simulink model "sim_battery_pack_simulink_18_11"  (R2021a)
settings: Solver=FixedStepAuto  StartTime=0.0  StopTime=3460.480  FixedStep=0.01  RelTol=1e-3
values from neighbouring files (symbols this model uses):
  Af = 1.4*1.6    (= 2.24)    [battery_pack_init_18_11.m]
  b = 0.002    [battery_pack_init_18_11.m]
  Batt_Eff = .98    (= 0.98)    [battery_pack_init_18_11.m]
  Batt_Ene_Cap = 7.37    [battery_pack_init_18_11.m]
  cd = 0.45    [battery_pack_init_18_11.m]
  dt = 0.01    [battery_pack_init_18_11.m]
  g = 9.81    [battery_pack_init_18_11.m]
  Gr = 5.75*.85    (= 4.8875)    [battery_pack_init_18_11.m]
  Grade = 7    [battery_pack_init_18_11.m]
  Ini_SOC = 100    [battery_pack_init_18_11.m]
  kappa = 0.1    [battery_pack_init_18_11.m]
  M = M_k+M_P    (= 445)    [battery_pack_init_18_11.m]
  M_Trq = T_m    [battery_pack_init_18_11.m]
  M_w = w_m    [battery_pack_init_18_11.m]
  Mot_Eff = .9    (= 0.9)    [battery_pack_init_18_11.m]
  mu = 0.016    [battery_pack_init_18_11.m]
  Np = 7    [battery_pack_init_18_11.m]
  Ns = 12    [battery_pack_init_18_11.m]
  Qgain = 1    [battery_pack_init_18_11.m]
  R0 = zeros(numpoles,1)    [battery_pack_init_18_11.m]
  R0Param = getParamESC('R0Param',T,cell_model)    [battery_pack_init_18_11.m]
  R_w = .3048/2    (= 0.1524)    [battery_pack_init_18_11.m]
  Re_spe_max = 50*5/18    (= 13.8888888889)    [battery_pack_init_18_11.m]
  Re_spe_min = 0*5/18    (= 0)    [battery_pack_init_18_11.m]
  rho = 1.225    [battery_pack_init_18_11.m]
  rt = .0008    (= 0.0008)    [battery_pack_init_18_11.m]
  T = 40    [battery_pack_init_18_11.m]
  T_MIDC = T_MIDC(1:72)    [battery_pack_init_18_11.m]
  Trans_Eff = .95    (= 0.95)    [battery_pack_init_18_11.m]
  V_MIDC = V_MIDC(1:72)    [battery_pack_init_18_11.m]
  Z0 = 0.75 + (1-0.75).*rand(1,Np)    [battery_pack_init_18_11.m]
undefined symbols (not defined in the file or in its folder): cell_model, FLbattery, gain, iload, sigbuilder_block, VMIDC
libraries: simulink x16, autolibshared x2, pid_lib x1, simulink_extras x1
(part 3 of 17)

== system sim_battery_pack_simulink_18_11/SCM7/cell6 ==
  ik1 : Inport
  Constant : Constant  Value=R0
  Constant1 : Constant  Value=dt
  Constant2 : Constant  Value=T
  States : Scope  NumInputPorts=2
  Unit Delay : UnitDelay  InitialCondition=Z0(6,7)  SampleTime=-1  HasFrameUpgradeWarning=on
  Unit Delay1 : UnitDelay  SampleTime=-1  HasFrameUpgradeWarning=on
  Voltage : Scope  NumInputPorts=2
  cell_model : MATLAB Function  TreatAsAtomicUnit=on
  V1 : Outport
  Z1 : Outport  Port=2
  irc1 : Outport  Port=3
  wires:
  cell_model/4(OCV) -> Voltage/2
  ik1/1 -> cell_model/6(ik)
  cell_model/3(zkc) -> Z1/1, Unit Delay/1, States/1
  cell_model/1(vk) -> V1/1, Voltage/1
  Constant1/1 -> cell_model/2(deltaT)
  Constant2/1 -> cell_model/1(T)
  Unit Delay/1 -> cell_model/4(zkp)
  cell_model/2(irkc) -> irc1/1, Unit Delay1/1, States/2
  Unit Delay1/1 -> cell_model/5(irkp)
  Constant/1 -> cell_model/3(iR0)

== system sim_battery_pack_simulink_18_11/SCM7/cell7 ==
  ik1 : Inport
  Constant : Constant  Value=R0
  Constant1 : Constant  Value=dt
  Constant2 : Constant  Value=T
  States : Scope  NumInputPorts=2
  Unit Delay : UnitDelay  InitialCondition=Z0(7,7)  SampleTime=-1  HasFrameUpgradeWarning=on
  Unit Delay1 : UnitDelay  SampleTime=-1  HasFrameUpgradeWarning=on
  Voltage : Scope  NumInputPorts=2
  cell_model : MATLAB Function  TreatAsAtomicUnit=on
  V1 : Outport
  Z1 : Outport  Port=2
  irc1 : Outport  Port=3
  wires:
  Constant/1 -> cell_model/3(iR0)
  Unit Delay1/1 -> cell_model/5(irkp)
  cell_model/2(irkc) -> States/2, Unit Delay1/1, irc1/1
  Unit Delay/1 -> cell_model/4(zkp)
  Constant2/1 -> cell_model/1(T)
  Constant1/1 -> cell_model/2(deltaT)
  cell_model/1(vk) -> Voltage/1, V1/1
  cell_model/3(zkc) -> States/1, Unit Delay/1, Z1/1
  ik1/1 -> cell_model/6(ik)
  cell_model/4(OCV) -> Voltage/2

== system sim_battery_pack_simulink_18_11/SCM7/cell8 ==
  ik1 : Inport
  Constant : Constant  Value=R0
  Constant1 : Constant  Value=dt
  Constant2 : Constant  Value=T
  States : Scope  NumInputPorts=2
  Unit Delay : UnitDelay  InitialCondition=Z0(8,7)  SampleTime=-1  HasFrameUpgradeWarning=on
  Unit Delay1 : UnitDelay  SampleTime=-1  HasFrameUpgradeWarning=on
  Voltage : Scope  NumInputPorts=2
  cell_model : MATLAB Function  TreatAsAtomicUnit=on
  V1 : Outport
  Z1 : Outport  Port=2
  irc1 : Outport  Port=3
  wires:
  cell_model/4(OCV) -> Voltage/2
  ik1/1 -> cell_model/6(ik)
  cell_model/3(zkc) -> Z1/1, Unit Delay/1, States/1
  cell_model/1(vk) -> V1/1, Voltage/1
  Constant1/1 -> cell_model/2(deltaT)
  Constant2/1 -> cell_model/1(T)
  Unit Delay/1 -> cell_model/4(zkp)
  cell_model/2(irkc) -> irc1/1, Unit Delay1/1, States/2
  Unit Delay1/1 -> cell_model/5(irkp)
  Constant/1 -> cell_model/3(iR0)

== system sim_battery_pack_simulink_18_11/SCM7/cell9 ==
  ik1 : Inport
  Constant : Constant  Value=R0
  Constant1 : Constant  Value=dt
  Constant2 : Constant  Value=T
  States : Scope  NumInputPorts=2
  Unit Delay : UnitDelay  InitialCondition=Z0(9,7)  SampleTime=-1  HasFrameUpgradeWarning=on
  Unit Delay1 : UnitDelay  SampleTime=-1  HasFrameUpgradeWarning=on
  Voltage : Scope  NumInputPorts=2
  cell_model : MATLAB Function  TreatAsAtomicUnit=on
  V1 : Outport
  Z1 : Outport  Port=2
  irc1 : Outport  Port=3
  wires:
  Constant/1 -> cell_model/3(iR0)
  Unit Delay1/1 -> cell_model/5(irkp)
  cell_model/2(irkc) -> States/2, Unit Delay1/1, irc1/1
  Unit Delay/1 -> cell_model/4(zkp)
  Constant2/1 -> cell_model/1(T)
  Constant1/1 -> cell_model/2(deltaT)
  cell_model/1(vk) -> Voltage/1, V1/1
  cell_model/3(zkc) -> States/1, Unit Delay/1, Z1/1
  ik1/1 -> cell_model/6(ik)
  cell_model/4(OCV) -> Voltage/2

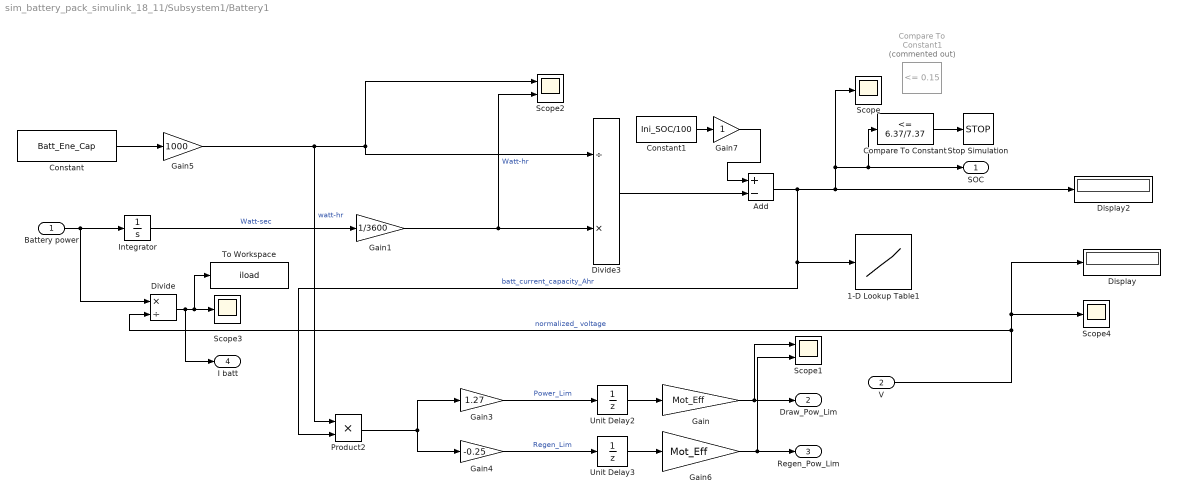
== system sim_battery_pack_simulink_18_11/Subsystem1/Battery1 ==
  Battery power : Inport
  V : Inport  Port=2
  1-D Lookup Table1 : Lookup_n-D  NumberOfTableDimensions=1  BreakpointsForDimension1=[0,0.01,0.02,0.03,0.04,0.05,0.06,0.07,0.08,0.09,0.1,0.11,0.12,0.13,0.14,0.15,0.16,0.17,0.18,0.19,0.2,0.21,0.22,0.23,0.24,0.25,0.26,0.27,0.28,0.29,0.3,0.31,0.32,0.33,0.34,0.35,0.36,0.37,0.38,0.39,0.4,0.41,0.42,0.43,0.44,0.45,0.46,0.47,0.48,0.49,0.5,0.51,0.52,0.53,0.54,0.55,0.56,0.57,0.58,0.59,0.6,0.61,0.62,0.63,0.64,0.65,0.66,0.67,0.68,0.69,0.7,0.71,0.72,0.73,0.74,0.75,0.76,0.77,0.78,0.79,0.8,0.81,0.82,0.83,0.84,0.85,0.86,0.87,0.88,0.89,0.9,0.91,0.92,0.93,0.94,0.95,0.96,0.97,0.98,0.99,1]  Table=[31.919999999999998,36.799200000000006,37.437599999999996,38.315400000000004,38.8512,39.0678,39.5808,39.6378,39.8202,39.9456,40.0824,40.2192,40.3218,40.3195,40.5751,40.5112,40.5751,40.766400000000004,40.8918,40.9146,41.0224,41.04,41.1312,41.153999999999996,41.2224,41.256600000000006,41.3364,41.4048,41.461800000000004,41.496,41.5974,41.5644,41.6328,41.667,41.7012,41.7354,41.769600000000004,41.815200000000004,41.8722,41.9292,41.952000000000005,41.9634,42.0204,42.088800000000006,42.1686,42.2028,42.237,42.294000000000004,42.3738,42.4422,42.4992,42.6837,42.579,42.6198,42.738600000000005,42.807,42.875400000000006,42.9552,43.0122,43.092,43.1949,43.297200000000004,43.297200000000004,43.479600000000005,43.525200000000005,43.605000000000004,43.787400000000005,43.8444,43.947,44.0382,44.1978,44.289,44.391600000000004,44.5398,44.6766,44.756400000000006,44.859,44.961600000000004,45.0756,45.1896,45.3036,45.4632,45.577200000000005,45.759600000000006,45.9306,45.9876,46.135799999999996,46.34100000000001,46.443599999999996,46.580400000000004,46.7058,47.0934,47.03640000000001,47.1732,47.31,47.652,47.583600000000004,47.73180000000001,47.9598,48.2334,48.119400000000006]  ExtrapMethod=Clip  UseLastTableValue=on  InternalRulePriority=Speed  RndMeth=Simplest  InputSameDT=on
  Add : Sum  Inputs=+-
  Compare To Constant : simulink/Logic and Bit Operations/Compare To Constant  relop=<=  const=6.37/7.37  OutDataTypeStr=boolean
  Compare To Constant1 : simulink/Logic and Bit Operations/Compare To Constant  Commented=on  relop=<=  const=0.15  OutDataTypeStr=boolean
  Constant : Constant  Value=Batt_Ene_Cap
  Constant1 : Constant  Value=Ini_SOC/100
  Display : Display
  Display2 : Display
  Divide : Product  Inputs=*/
  Divide3 : Product  Inputs=/*
  Gain : Gain  Gain=Mot_Eff
  Gain1 : Gain  Gain=1/3600
  Gain3 : Gain  Gain=1.27
  Gain4 : Gain  Gain=-0.25
  Gain5 : Gain  Gain=1000
  Gain6 : Gain  Gain=Mot_Eff
  Gain7 : Gain
  Integrator : Integrator
  Product2 : Product
  Scope : Scope
  Scope1 : Scope  NumInputPorts=2
  Scope2 : Scope  NumInputPorts=2
  Scope3 : Scope
  Scope4 : Scope
  Stop Simulation : Stop
  To Workspace : ToWorkspace  VariableName=iload  SampleTime=-1
  Unit Delay2 : UnitDelay  SampleTime=-1  HasFrameUpgradeWarning=on
  Unit Delay3 : UnitDelay  SampleTime=-1  HasFrameUpgradeWarning=on
  SOC : Outport
  Draw_Pow_Lim : Outport  Port=2
  Regen_Pow_Lim : Outport  Port=3
  I batt : Outport  Port=4
  wires:
  Constant/1 -> Gain5/1
  Integrator/1 -> Gain1/1  "Watt-sec"
  Add/1 -> Compare To Constant/1, SOC/1, Scope/1, Display2/1, 1-D Lookup Table1/1, Product2/2  "batt_current_capacity_Ahr"
  Compare To Constant/1 -> Stop Simulation/1
  V/1 -> Display/1, Scope4/1, Divide/2  "normalized_ voltage"
  Gain3/1 -> Unit Delay2/1  "Power_Lim"
  Gain4/1 -> Unit Delay3/1  "Regen_Lim"
  Gain1/1 -> Scope2/2, Divide3/2  "Watt-hr"
  Divide3/1 -> Add/2
  Gain7/1 -> Add/1
  Product2/1 -> Gain4/1, Gain3/1
  Gain6/1 -> Regen_Pow_Lim/1, Scope1/2
  Constant1/1 -> Gain7/1
  Gain5/1 -> Product2/1, Divide3/1, Scope2/1  "watt-hr"
  Battery power/1 -> Divide/1, Integrator/1
  Unit Delay2/1 -> Gain/1
  Unit Delay3/1 -> Gain6/1
  Gain/1 -> Draw_Pow_Lim/1, Scope1/1
  Divide/1 -> I batt/1, To Workspace/1, Scope3/1

== system sim_battery_pack_simulink_18_11/Subsystem1/Controller ==
  AccelCmd : Inport
  Brake : Inport  Port=2
  VehSpd : Inport  Port=3
  Draw_Lim : Inport  Port=4
  Regen_Lim : Inport  Port=5
  MtrSpd : Inport  Port=6
  Controller : Subsystem
  Scope : Scope  NumInputPorts=3
  Subsystem : Subsystem
  TrqCmd : Outport
  BrkForce : Outport  Port=2
  tag scope: BrkPrs=global, TrqCmd=global
  wires:
  Brake/1 -> Controller/2(Brake)
  [MtrSpd] -> Controller/3(MotSpd)  "mtr_spd"
  VehSpd/1 -> Controller/5(VehSpd)
  [Soc] -> Controller/4(SOC)  "batt_SOC"
  Controller/2(Brkprs) -> Scope/3, BrkForce/1, [BrkPrs]  "controller_brkforce"
  Controller/1(TrqCmd) -> Subsystem/4(controller_trqcmd), Scope/2, [TrqCmd]  "controller_trqcmd"
  AccelCmd/1 -> Controller/1(AccelCmd)
  Draw_Lim/1 -> Subsystem/1(Draw_pow_lim)
  MtrSpd/1 -> Subsystem/2(Motor_Speed)
  Regen_Lim/1 -> Subsystem/3(Regen_Pow_Lim)
  Subsystem/1(y) -> Scope/1, TrqCmd/1

== system sim_battery_pack_simulink_18_11/Subsystem1/Driver ==
  VelFdbk : Inport
  1-D Lookup Table : Lookup_n-D  NumberOfTableDimensions=1  BreakpointsForDimension1=[T_MIDC]  Table=[V_MIDC]  InternalRulePriority=Speed  RndMeth=Simplest  InputSameDT=on
  Abs : Abs
  Clock : Clock
  Compare To Constant : simulink/Logic and Bit Operations/Compare To Constant  relop=>=  const=0  OutDataTypeStr=boolean
  Compare To Constant1 : simulink/Logic and Bit Operations/Compare To Constant  relop=<  const=0  OutDataTypeStr=boolean
  Constant1 : Constant
  Constant2 : Constant  Value=773
  Constant3 : Constant  Value=0
  Drive Cycle Source : autolibshared/Drive Cycle Source  cycleVar=Japanese 10-15 Mode  wsVar=[T_MIDC,VMIDC]  fileVar=cycleFTP75.mat  tfinal="660  seconds, Cyclic"  cycleRepeat=on  outAccPort=off  outGearPort=off  gearList=No gear data  t_wot1=5  xdot_woto=0  xdot_wot1=30  t_wot2=20  xdot_wot2=0  t_wotend=30  srcUnit=m/s  outUnit=km/h  srcAccUnit=m/s/s  outAccUnit=m/s^2  dt=0  aMode=1  faultOption=off  velBnd=2  velBndUnit=mph  inUnit=m/s  timeBnd=1  failOption=off  stopSim=off  maxFaultCnt=10  maxFaultTime=2  maxTotFaultTime=15  traceOption=off  dtTrace=1  traceWindow=10  lastDCname=Japanese 10-15 Mode  lastOutUnit=mph  lastDT=0  lastTB=1  lastSB=2  forceCalcBound=off
      settings: SourceProductBaseCode=PW,DR,MT,UV,VE
  Gain4 : Gain  Gain=5/18
  Mod : Math  Operator=mod  SaturateOnIntegerOverflow=on
  PID Controller : pid_lib/PID Controller  Controller=PID  Form=Parallel  TimeDomain=Continuous-time  UseExternalTs=off  SampleTime=-1  IntegratorMethod=Forward Euler  FilterMethod=Forward Euler  ControllerParametersSource=internal  P=1.2  I=.1  D=.1  UseFilter=on  N=100  TunerSelectOption=Transfer Function Based (PID Tuner App)  InitialConditionSource=internal  InitialConditionForIntegrator=0  InitialConditionForFilter=0  DifferentiatorICPrevScaledInput=0  ExternalReset=none  TrackingMode=off  Kt=1  LimitOutput=on  SatLimitsSource=internal  UpperSaturationLimit=1  LowerSaturationLimit=-1  LinearizeAsGain=on  AntiWindupMode=clamping  Kb=1  POutMin=[]  POutMax=[]  IOutMin=[]  IOutMax=[]  DOutMin=[]  DOutMax=[]  NOutMin=[]  NOutMax=[]  SumOutMin=[]  SumOutMax=[]  SaturationOutMin=[]  SaturationOutMax=[]  PParamMin=[]  PParamMax=[]  IParamMin=[]  IParamMax=[]  DParamMin=[]  DParamMax=[]  NParamMin=[]  NParamMax=[]  KbParamMin=[]  KbParamMax=[]  KtParamMin=[]  KtParamMax=[]  KbOutMin=[]  KbOutMax=[]  KtOutMin=[]  KtOutMax=[]  IntegratorOutMin=[]  IntegratorOutMax=[]  FilterOutMin=[]  FilterOutMax=[]  SumI1OutMin=[]  SumI1OutMax=[]  SumI2OutMin=[]  SumI2OutMax=[]  SumI3OutMin=[]  SumI3OutMax=[]  SumI4OutMin=[]  SumI4OutMax=[]  SumDOutMin=[]  SumDOutMax=[]  DifferentiatorOutMin=[]  DifferentiatorOutMax=[]  FilterDiffOutCoefMin=[]  FilterDiffOutCoefMax=[]  ReciprocalOutMin=[]  ReciprocalOutMax=[]  SumDenOutMin=[]  SumDenOutMax=[]  SumNumOutMin=[]  SumNumOutMax=[]  DivideOutMin=[]  DivideOutMax=[]  UdiffTsProdOutMin=[]  UdiffTsProdOutMax=[]  NTsProdOutMin=[]  NTsProdOutMax=[]  UintegralTsProdOutMin=[]  UintegralTsProdOutMax=[]  UngainTsProdOutMin=[]  UngainTsProdOutMax=[]  IntegratorContinuousStateAttributes=''  IntegratorStateMustResolveToSignalObject=off  IntegratorRTWStateStorageClass=Auto  FilterContinuousStateAttributes=''  FilterStateMustResolveToSignalObject=off  FilterRTWStateStorageClass=Auto  ParallelPVariant=InternalParameters  IdealPVariant=Disabled  IVariant=InternalParameters  DVariant=InternalParameters  IntegratorVariant=Continuous  SatVariant=Enabled  AWVariant=ContClampingParallel  PCopyVariant=Disabled  TRVariant=Disabled  FdbkBlocksVariant=Forward  IdealPFdbkVariant=Disabled  SatFdbkVariant=Disabled  DerivativeFilterVariant=ContFilter  NVariant=InternalParameters  NCopyVariant=Disabled  FilterICVariant=InternalICsFilter  IntegratorICVariant=InternalICs  ExternalResetVariant=Disabled  TRSumVariant=Passthrough  SumFdbkVariant=Disabled  SumVariant=Sum_PID  TsampFilterVariant=InternalTs  TsampNgainVariant=Passthrough  TsampIntegralVariant=Passthrough  ExternalSaturationOutDataTypeStr=Inherit: Same as second input
  Product : Product
  Product1 : Product
  Scope : Scope  NumInputPorts=2
  Signal Builder1 : Subsystem  Tag=STV Subsys  Commented=on  LoadFcn=sigbuilder_block('load');  StartFcn=sigbuilder_block('start');  StopFcn=sigbuilder_block('stop');  ClipboardFcn=sigbuilder_block('clipboard');  mask(Sigbuilder block){tuvar=[0:10]}
      mask help: Simulink:masks:SigbuilderBlock_MD
      mask init:
      | if ~strcmp(get_param(bdroot(gcbh),'SimulationStatus'),'stopped') tuvar = sigbuilder_block('maskInit'); end
      settings: CopyFcn=sigbuilder_block('copy');  DeleteFcn=sigbuilder_block('delete');  ModelCloseFcn=sigbuilder_block('modelClose');  PreSaveFcn=sigbuilder_block('preSave');  PauseFcn=sigbuilder_block('pause');  ContinueFcn=sigbuilder_block('continue');  NameChangeFcn=sigbuilder_block('namechange');  OpenFcn=sigbuilder_block('open',[437.6 153 550.4 359.25 ]);  CloseFcn=sigbuilder_block('close');
      mask Display: plot(0, 0, 100, 100,[2, 2, 32, 32, 2], [68, 8, 8, 68, 68],[32, 2], [38, 38], [32, 19, 2],[53, 60, 44], [32, 17, 17, 2],[16, 16, 31, 31]);txt = getActiveGroup(gcbh);text(2, 100, txt,'verticalAlignment', 'top');
  Sum : Sum  Inputs=|+-
  AccelCmd : Outport
  DecelCmd : Outport  Port=2
  Vref : Outport  Port=3
  tag scope: RefSpd=global
  wires:
  Gain4/1 -> [RefSpd], Sum/1  "m/s"
  VelFdbk/1 -> Sum/2
  Product1/1 -> DecelCmd/1, Scope/2  "brk_cmd"
  Sum/1 -> PID Controller/1
  Compare To Constant/1 -> Product/2
  Compare To Constant1/1 -> Product1/2
  PID Controller/1 -> Compare To Constant1/1, Abs/1, Compare To Constant/1, Product/1
  Abs/1 -> Product1/1
  Clock/1 -> Mod/1
  Constant2/1 -> Mod/2
  Mod/1 -> 1-D Lookup Table/1
  1-D Lookup Table/1 -> Gain4/1, Vref/1  "acc_cmd"
  Product/1 -> AccelCmd/1, Scope/1  "acc_cmd"

== system sim_battery_pack_simulink_18_11/Subsystem1/Motor ==
  TrqCmd : Inport
  MtrSpd : Inport  Port=2
  1-D Lookup Table : Lookup_n-D  NumberOfTableDimensions=1  BreakpointsForDimension1=M_w  Table=M_Trq  ExtrapMethod=Clip  UseLastTableValue=on  InternalRulePriority=Speed  RndMeth=Simplest  InputSameDT=on
  1-D Lookup Table1 : Lookup_n-D  NumberOfTableDimensions=1  BreakpointsForDimension1=M_w  Table=-M_Trq*0.5  ExtrapMethod=Clip  UseLastTableValue=on  InternalRulePriority=Speed  RndMeth=Simplest  InputSameDT=on
  Compare To Constant : simulink/Logic and Bit Operations/Compare To Constant  relop=>=  const=1  OutDataTypeStr=boolean
  Constant : Constant  Value=Batt_Eff
  Gain : Gain  Gain=1/Mot_Eff
  Gain1 : Gain  Gain=b
  KW : Gain  Gain=.001
  Min : MinMax  Inputs=2
  Min1 : MinMax  Function=max  Inputs=2
  Product : Product  Inputs=**
  Product1 : Product  Inputs=**
  Product2 : Product
  Scope : Scope  NumInputPorts=3
  Scope1 : Scope  NumInputPorts=3
  Scope2 : Scope  NumInputPorts=2
  Scope3 : Scope  NumInputPorts=2
  Scope4 : Scope
  Subtract : Sum  Inputs=+-
  Switch : Switch  Criteria=u2 > Threshold
  Switch1 : Switch  Criteria=u2 > Threshold
  Batt_Pow_Cons : Outport
  Mtr_trq : Outport  Port=2
  wires:
  TrqCmd/1 -> Scope3/2, Scope2/2, Min1/2, Switch1/2, Switch/2, Min/2
  Switch/1 -> Scope/1, Scope1/1, Subtract/1, Product/1
  MtrSpd/1 -> Gain1/1, Compare To Constant/1, Scope/2, Product/2, 1-D Lookup Table/1, 1-D Lookup Table1/1
  Product/1 -> Switch1/1, Product1/1, KW/1  "Mot mech power"
  1-D Lookup Table/1 -> Scope3/1, Min/1
  Product2/1 -> Scope1/2, Subtract/2
  Subtract/1 -> Scope1/3, Mtr_trq/1
  Compare To Constant/1 -> Product2/2
  Gain1/1 -> Product2/1
  Gain/1 -> Scope4/1, Batt_Pow_Cons/1  "batt_Pow"
  1-D Lookup Table1/1 -> Scope2/1, Min1/1
  Min1/1 -> Switch/3
  Min/1 -> Switch/1
  Switch1/1 -> Gain/1
  Product1/1 -> Switch1/3  "Mot mech power"
  Constant/1 -> Product1/2
  KW/1 -> Scope/3

== system sim_battery_pack_simulink_18_11/Subsystem1/Transmission ==
  MtrTrq : Inport
  AxleSpd : Inport  Port=2
  Gain : Gain  Gain=Gr
  Gain1 : Gain  Gain=Gr
  Gain2 : Gain  Gain=Trans_Eff
  Product : Product
  Scope : Scope
  AxleTrq : Outport
  MtrSpd : Outport  Port=2
  tag scope: MtrSpd=global
  wires:
  Gain/1 -> Product/2, AxleTrq/1  "singlemotorunit_mtrtrq"
  Gain1/1 -> MtrSpd/1, [MtrSpd]  "mtr_spd_radps"
  Product/1 -> Scope/1
  Gain2/1 -> Gain/1
  AxleSpd/1 -> Gain1/1, Product/1
  MtrTrq/1 -> Gain2/1

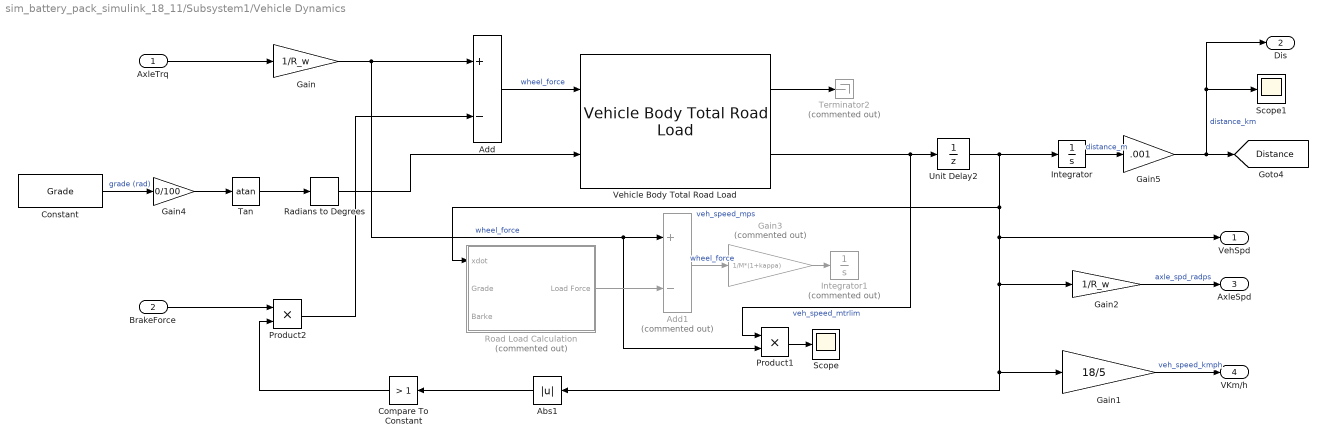
== system sim_battery_pack_simulink_18_11/Subsystem1/Vehicle Dynamics ==
  AxleTrq : Inport
  BrakeForce : Inport  Port=2
  Abs1 : Abs
  Add : Sum  Inputs=+-
  Add1 : Sum  Commented=on  Inputs=+-
  Compare To Constant : simulink/Logic and Bit Operations/Compare To Constant  relop=>  const=1  OutDataTypeStr=boolean
  Constant : Constant  Value=Grade
  Gain : Gain  Gain=1/R_w
  Gain1 : Gain  Gain=18/5
  Gain2 : Gain  Gain=1/R_w
  Gain3 : Gain  Commented=on  Gain=1/M*(1+kappa)
  Gain4 : Gain  Gain=0/100
  Gain5 : Gain  Gain=.001
  Integrator : Integrator
  Integrator1 : Integrator  Commented=on
  Product1 : Product
  Product2 : Product
  Radians to Degrees : simulink_extras/Transformations/Radians to Degrees
  Road Load Calculation : Subsystem  Commented=on
  Scope : Scope
  Scope1 : Scope
  Tan : Trigonometry  Operator=atan
  Terminator2 : Terminator  Commented=on
  Unit Delay2 : UnitDelay  SampleTime=-1  HasFrameUpgradeWarning=on
  Vehicle Body Total Road Load : autolibshared/Vehicle Body Total Road Load  VariantControl=SL1dof  input_type=Force  aMode=1  m=M  a=M*g*mu  b=0/R_w^2  c=0.5*cd*rho*Af  g=g  x_o=0  xdot_o=0
      settings: SourceProductBaseCode=PW,DR,MT,UV,VE
  VehSpd : Outport
  Dis : Outport  Port=2
  AxleSpd : Outport  Port=3
  VKm/h : Outport  Port=4
  tag scope: Distance=global
  wires:
  Gain/1 -> Add/1, Product1/2, Add1/1  "wheel_force"
  Tan/1 -> Radians to Degrees/1
  Vehicle Body Total Road Load/1 -> Terminator2/1
  Integrator/1 -> Gain5/1  "distance_m"
  Product2/1 -> Add/2
  Gain5/1 -> Scope1/1, Dis/1, [Distance]  "distance_km"
  AxleTrq/1 -> Gain/1
  Gain2/1 -> AxleSpd/1  "axle_spd_radps"
  Gain1/1 -> VKm/h/1  "veh_speed_kmph"
  Vehicle Body Total Road Load/2 -> Unit Delay2/1, Product1/1  "veh_speed_mtrlim"
  Road Load Calculation/1(Load Force) -> Add1/2
  Add1/1 -> Gain3/1  "wheel_force"
  Gain3/1 -> Integrator1/1
  Product1/1 -> Scope/1
  Radians to Degrees/1 -> Vehicle Body Total Road Load/2
  Add/1 -> Vehicle Body Total Road Load/1  "wheel_force"
  BrakeForce/1 -> Product2/1
  Compare To Constant/1 -> Product2/2
  Abs1/1 -> Compare To Constant/1
  Constant/1 -> Gain4/1  "grade (rad)"
  Gain4/1 -> Tan/1
  Unit Delay2/1 -> VehSpd/1, Abs1/1, Gain1/1, Gain2/1, Road Load Calculation/1(xdot), Integrator/1  "veh_speed_mps"

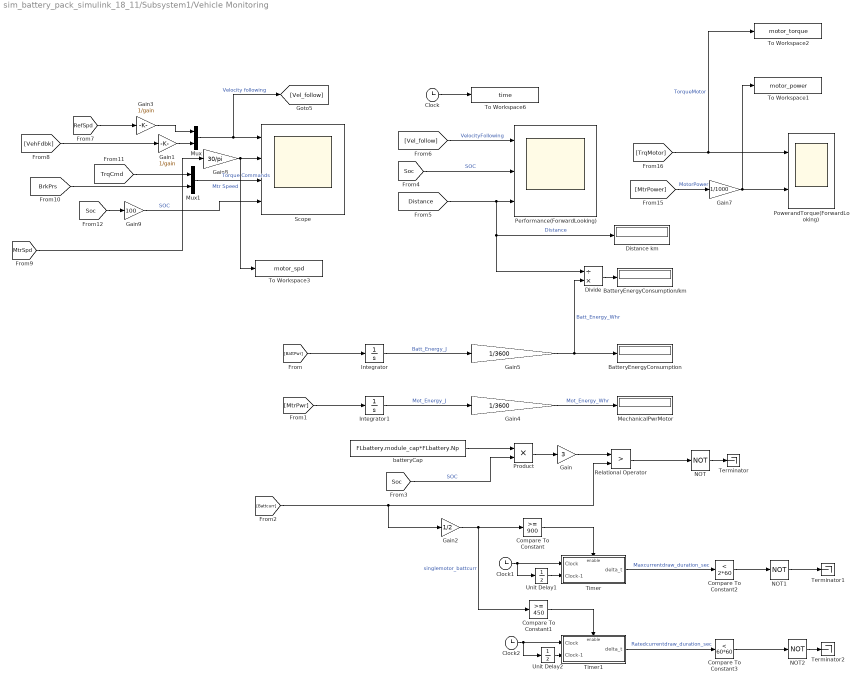
== system sim_battery_pack_simulink_18_11/Subsystem1/Vehicle Monitoring ==
  BatteryEnergyConsumption : Display
  BatteryEnergyConsumption/km : Display
  Clock : Clock
  Clock1 : Clock
  Clock2 : Clock
  Compare To Constant : simulink/Logic and Bit Operations/Compare To Constant  relop=>=  const=900  OutDataTypeStr=boolean
  Compare To Constant1 : simulink/Logic and Bit Operations/Compare To Constant  relop=>=  const=450  OutDataTypeStr=boolean
  Compare To Constant2 : simulink/Logic and Bit Operations/Compare To Constant  relop=<  const=2*60  OutDataTypeStr=boolean
  Compare To Constant3 : simulink/Logic and Bit Operations/Compare To Constant  relop=<  const=60*60  OutDataTypeStr=boolean
  Distance km : Display
  Divide : Product  Inputs=/*
  Gain : Gain  Gain=3
  Gain1 : Gain  Gain=1/gain
  Gain2 : Gain  Gain=1/2
  Gain3 : Gain  Gain=1/gain
  Gain4 : Gain  Gain=1/3600
  Gain5 : Gain  Gain=1/3600
  Gain7 : Gain  Gain=1/1000
  Gain8 : Gain  Gain=30/pi
  Gain9 : Gain  Gain=100
  Integrator : Integrator
  Integrator1 : Integrator
  MechanicalPwrMotor : Display
  Mux : Mux  Inputs=2
  Mux1 : Mux  Inputs=2
  NOT : Logic  Operator=NOT  IconShape=distinctive  AllPortsSameDT=off  OutDataTypeStr=boolean
  NOT1 : Logic  Operator=NOT  IconShape=distinctive  AllPortsSameDT=off  OutDataTypeStr=boolean
  NOT2 : Logic  Operator=NOT  IconShape=distinctive  AllPortsSameDT=off  OutDataTypeStr=boolean
  Performance(ForwardLooking) : Scope  NumInputPorts=3
  PowerandTorque(ForwardLooking) : Scope  NumInputPorts=2
  Product : Product
  Relational Operator : RelationalOperator  Operator=>  OutDataTypeStr=boolean  RndMeth=Simplest
  Scope : Scope  NumInputPorts=4
  Terminator : Terminator
  Terminator1 : Terminator
  Terminator2 : Terminator
  Timer : Subsystem  TreatAsAtomicUnit=on
  Timer1 : Subsystem  TreatAsAtomicUnit=on
  To Workspace1 : ToWorkspace  VariableName=motor_power  SampleTime=-1
      settings: Save2DSignal=2-D array (concatenate along first dimension)
  To Workspace2 : ToWorkspace  VariableName=motor_torque  SampleTime=-1
      settings: Save2DSignal=2-D array (concatenate along first dimension)
  To Workspace3 : ToWorkspace  VariableName=motor_spd  SampleTime=-1
      settings: Save2DSignal=2-D array (concatenate along first dimension)
  To Workspace6 : ToWorkspace  VariableName=time  SampleTime=-1
      settings: Save2DSignal=2-D array (concatenate along first dimension)
  Unit Delay1 : UnitDelay  SampleTime=-1  HasFrameUpgradeWarning=on
  Unit Delay2 : UnitDelay  SampleTime=-1  HasFrameUpgradeWarning=on
  batteryCap : Constant  Value=FLbattery.module_cap*FLbattery.Np
  wires:
  Gain1/1 -> Mux/2
  Mux/1 -> [Vel_follow], Scope/1  "Velocity following"
  Clock/1 -> To Workspace6/1
  [Vel_follow] -> Performance(ForwardLooking)/1  "VelocityFollowing"
  [BrkPrs] -> Mux1/2
  [TrqMotor] -> To Workspace2/1, PowerandTorque(ForwardLooking)/1  "TorqueMotor"
  [RefSpd] -> Gain3/1
  [MtrSpd] -> Gain8/1
  Gain8/1 -> To Workspace3/1, Scope/2  "Mtr Speed"
  [TrqCmd] -> Mux1/1
  [MtrPower] -> Gain7/1  "MotorPower"
  Gain3/1 -> Mux/1
  Mux1/1 -> Scope/3  "Torque Commands"
  [Soc] -> Gain9/1
  [Soc] -> Performance(ForwardLooking)/2  "SOC"
  [Distance] -> Divide/1, Distance km/1, Performance(ForwardLooking)/3  "Distance"
  Gain7/1 -> To Workspace1/1, PowerandTorque(ForwardLooking)/2
  [VehFdbk] -> Gain1/1
  Gain9/1 -> Scope/4  "SOC"
  [BattPwr] -> Integrator/1
  Integrator/1 -> Gain5/1  "Batt_Energy_J"
  Gain5/1 -> Divide/2, BatteryEnergyConsumption/1  "Batt_Energy_Whr"
  Divide/1 -> BatteryEnergyConsumption/km/1
  [MtrPwr] -> Integrator1/1
  Integrator1/1 -> Gain4/1  "Mot_Energy_J"
  Gain4/1 -> MechanicalPwrMotor/1  "Mot_Energy_Whr"
  [Battcurr] -> Relational Operator/2, Gain2/1
  [Soc] -> Product/2  "SOC"
  batteryCap/1 -> Product/1
  Product/1 -> Gain/1
  Gain/1 -> Relational Operator/1
  Relational Operator/1 -> NOT/1
  Clock1/1 -> Unit Delay1/1, Timer/1(Clock)
  Unit Delay1/1 -> Timer/2(Clock-1)
  Compare To Constant/1 -> Timer/Enable
  Gain2/1 -> Compare To Constant1/1, Compare To Constant/1  "singlemotor_battcurr"
  Timer/1(delta_t) -> Compare To Constant2/1  "Maxcurrentdraw_duration_sec"
  Compare To Constant2/1 -> NOT1/1
  Unit Delay2/1 -> Timer1/2(Clock-1)
  Clock2/1 -> Unit Delay2/1, Timer1/1(Clock)
  Timer1/1(delta_t) -> Compare To Constant3/1  "Ratedcurrentdraw_duration_sec"
  Compare To Constant1/1 -> Timer1/Enable
  Compare To Constant3/1 -> NOT2/1
  NOT/1 -> Terminator/1
  NOT1/1 -> Terminator1/1
  NOT2/1 -> Terminator2/1

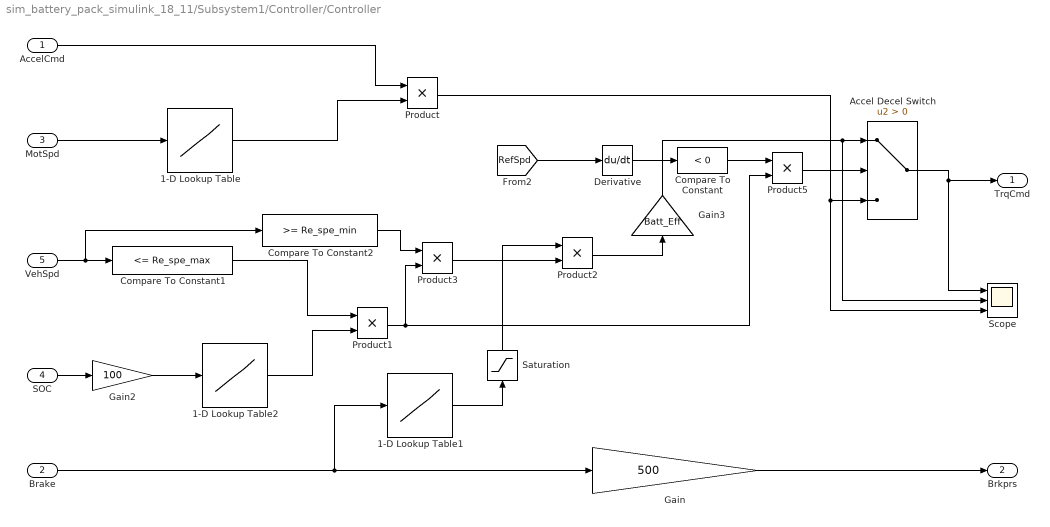
== system sim_battery_pack_simulink_18_11/Subsystem1/Controller/Controller ==
  AccelCmd : Inport
  Brake : Inport  Port=2
  MotSpd : Inport  Port=3
  SOC : Inport  Port=4
  VehSpd : Inport  Port=5
  1-D Lookup Table : Lookup_n-D  NumberOfTableDimensions=1  BreakpointsForDimension1=M_w  Table=M_Trq  ExtrapMethod=Clip  UseLastTableValue=on  InternalRulePriority=Speed  RndMeth=Simplest  InputSameDT=on
  1-D Lookup Table1 : Lookup_n-D  NumberOfTableDimensions=1  BreakpointsForDimension1=M_w  Table=-M_Trq*0.5  ExtrapMethod=Clip  UseLastTableValue=on  InternalRulePriority=Speed  RndMeth=Simplest  InputSameDT=on
  1-D Lookup Table2 : Lookup_n-D  NumberOfTableDimensions=1  BreakpointsForDimension1=[0:10:100]  Table=[1 1 1 1 1 1 1 0.7 0.5 0.2 0]  InternalRulePriority=Speed  OutDataTypeStr=double  RndMeth=Simplest  InputSameDT=on
  Accel Decel Switch : Switch  Criteria=u2 > Threshold
  Compare To Constant : simulink/Logic and Bit Operations/Compare To Constant  relop=<  const=0  OutDataTypeStr=boolean
  Compare To Constant1 : simulink/Logic and Bit Operations/Compare To Constant  relop=<=  const=Re_spe_max  OutDataTypeStr=boolean
  Compare To Constant2 : simulink/Logic and Bit Operations/Compare To Constant  relop=>=  const=Re_spe_min  OutDataTypeStr=boolean
  Derivative : Derivative
  Gain : Gain  Gain=500
  Gain2 : Gain  Gain=100
  Gain3 : Gain  Gain=Batt_Eff
  Product{,1..3,5} (5 alike) : Product
  Saturation : Saturate  UpperLimit=0  LowerLimit=-20
  Scope : Scope  NumInputPorts=3
  TrqCmd : Outport
  Brkprs : Outport  Port=2
  wires:
  VehSpd/1 -> Compare To Constant2/1, Compare To Constant1/1
  1-D Lookup Table/1 -> Product/2
  AccelCmd/1 -> Product/1
  Gain/1 -> Brkprs/1
  SOC/1 -> Gain2/1
  Compare To Constant1/1 -> Product1/1
  Product1/1 -> Product5/2, Product3/2
  MotSpd/1 -> 1-D Lookup Table/1
  Brake/1 -> 1-D Lookup Table1/1, Gain/1
  Derivative/1 -> Compare To Constant/1
  Gain2/1 -> 1-D Lookup Table2/1
  [RefSpd] -> Derivative/1
  Product2/1 -> Gain3/1
  Compare To Constant2/1 -> Product3/1
  Product3/1 -> Product2/2
  1-D Lookup Table2/1 -> Product1/2
  Compare To Constant/1 -> Product5/1
  Product5/1 -> Accel Decel Switch/2
  1-D Lookup Table1/1 -> Saturation/1
  Product/1 -> Scope/3, Accel Decel Switch/3
  Accel Decel Switch/1 -> TrqCmd/1, Scope/1
  Gain3/1 -> Scope/2, Accel Decel Switch/1
  Saturation/1 -> Product2/1

== system sim_battery_pack_simulink_18_11/Subsystem1/Controller/Subsystem ==
  Draw_pow_lim : Inport
  Motor_Speed : Inport  Port=2
  Regen_Pow_Lim : Inport  Port=3
  controller_trqcmd : Inport  Port=4
  Abs : Abs
  Add : Sum
  Constant : Constant
  Divide : Product  Inputs=*/
  Divide1 : Product  Inputs=*/
  Saturation Dynamic : simulink/Discontinuities/Saturation Dynamic  OutMin=[]  OutMax=[]  OutDataTypeStr=Inherit: Same as second input  OutDataType=fixdt(1, 16)  OutScaling=2^-10  DoSatur=off
  Scope1 : Scope  NumInputPorts=4
  Scope2 : Scope  NumInputPorts=2
  y : Outport
  wires:
  Constant/1 -> Add/1
  Divide/1 -> Scope1/1, Saturation Dynamic/1
  Divide1/1 -> Scope1/2, Saturation Dynamic/3
  Saturation Dynamic/1 -> Scope1/4, y/1
  controller_trqcmd/1 -> Saturation Dynamic/2, Scope1/3
  Draw_pow_lim/1 -> Divide/1, Scope2/1
  Regen_Pow_Lim/1 -> Scope2/2, Divide1/1
  Add/1 -> Divide1/2, Divide/2
  Abs/1 -> Add/2
  Motor_Speed/1 -> Abs/1

== system sim_battery_pack_simulink_18_11/Subsystem1/Driver/Signal Builder1 ==
  Demux : Demux  Tag=STV Demux  Outputs=1
      settings: DisplayOption=none
  FromWs : FromWorkspace  Tag=STV FromWs  VariableName=tuvar
      SigBuilderData=|
      | common.afterFinalStr = 'Extrapolate'
      | common.sampleTime = 0
      | dataSet.timeRange = [0 1500]
      | dataSet.name = 'Group 1'
      | sbobj.Groups.Name = 'Group 1'
      | sbobj.Groups.Signals.Name = 'Signal 1'
      | sbobj.Groups.Signals.XData = [0 1465 1500]
      | sbobj.Groups.Signals.YData = [0 28 28]
      | sbobj.Groups.TimeRange = [0 1500]
  Signal 1 : Outport  Tag=STV Outport
  wires:
  FromWs/1 -> Demux/1
  Demux/1 -> Signal 1/1

== system sim_battery_pack_simulink_18_11/Subsystem1/Vehicle Dynamics/Road Load Calculation ==
  xdot : Inport
  Grade : Inport  Port=2  Unit=%
  Barke : Inport  Port=3
  Abs : Abs
  Add : Sum  Inputs=++++
  Compare To Zero : simulink/Logic and Bit Operations/Compare To Zero  relop=>  OutDataTypeStr=boolean
  Cos : Trigonometry
  Cos1 : Trigonometry  Operator=cos
  Gain : Gain  Gain=0.5*cd*Af*rho
  Gain1 : Gain  Gain=M*g
  Gain2 : Gain  Gain=mu*M*g
  Math Function : Math  Operator=square  SaturateOnIntegerOverflow=on
  Product : Product
  Product1 : Product
  Product2 : Product
  Scope : Scope  NumInputPorts=4
  Sign : Signum
  Load Force : Outport
  wires:
  Cos/1 -> Gain1/1
  Cos1/1 -> Gain2/1
  Product/1 -> Gain/1
  Gain1/1 -> Add/2, Scope/2  "grade_force"
  Product1/1 -> Add/3, Scope/3
  Grade/1 -> Cos1/1, Cos/1
  Gain2/1 -> Product1/1  "roll_forrce"
  Compare To Zero/1 -> Product2/1, Product1/2
  Add/1 -> Load Force/1  "roadload_force"
  Math Function/1 -> Product/1
  Gain/1 -> Scope/1, Add/1  "aerodynamic_force"
  xdot/1 -> Abs/1, Math Function/1, Sign/1
  Sign/1 -> Product/2
  Product2/1 -> Scope/4, Add/4
  Abs/1 -> Compare To Zero/1
  Barke/1 -> Product2/2

== system sim_battery_pack_simulink_18_11/Subsystem1/Vehicle Monitoring/Timer ==
  Clock : Inport
  Clock-1 : Inport  Port=2
  Enable : EnablePort
  Add : Sum  Inputs=|+-
  Add1 : Sum  Inputs=|++
  Unit Delay1 : UnitDelay  SampleTime=-1  HasFrameUpgradeWarning=on
  delta_t : Outport
  wires:
  Clock/1 -> Add/1
  Add1/1 -> Unit Delay1/1, delta_t/1
  Clock-1/1 -> Add/2
  Add/1 -> Add1/1
  Unit Delay1/1 -> Add1/2

== system sim_battery_pack_simulink_18_11/Subsystem1/Vehicle Monitoring/Timer1 ==
  Clock : Inport
  Clock-1 : Inport  Port=2
  Enable : EnablePort
  Add : Sum  Inputs=|+-
  Add1 : Sum  Inputs=|++
  Unit Delay1 : UnitDelay  SampleTime=-1  HasFrameUpgradeWarning=on
  delta_t : Outport
  wires:
  Clock/1 -> Add/1
  Add1/1 -> Unit Delay1/1, delta_t/1
  Clock-1/1 -> Add/2
  Add/1 -> Add1/1
  Unit Delay1/1 -> Add1/2

== matlab function sim_battery_pack_simulink_18_11/SCM3/cell7/cell_model ==
  data: vk output size=1; T input; deltaT input; iR0 input; zkp input; irkp input; irkc output size=3; zkc output size=1; OCV output size=1; cell_model parameter; ik input; Qgain parameter

% function [vk,irk,hk,zk,sik,OCV] = simCell(ik,T,deltaT,model,z0,iR0,h0)
% 
% Simulates an ESC model for input current ik at temperature T
%
% Inputs:  ik - current, where (+) is discharge
%          T  - temperature (degC)
%      deltaT - sampling interval in data (s)
%       model - standard model structure
%          z0 - initial cell state of charge
%         iR0 - initial resistor currents as column vector
%          h0 - initial hysteresis state
% Outputs: vk - cell voltage for all timesteps
%         irk - resistor currents (in R-C branches) for all timesteps
%          hk - hysteresis states for all timesteps
%          zk - state of charge for all timesteps
%         sik - instantaneous hysteresis for all timesteps
%         OCV - open-circuit voltage for all timesteps

% Copyright (c) 2015 by Gregory L. Plett of the University of Colorado 
% Colorado Springs (UCCS). This work is licensed under a Creative Commons 
% Attribution-NonCommercial-ShareAlike 4.0 Intl. License, v. 1.0.
% It is provided "as is", without express or implied warranty, for 
% educational and informational purposes only.
%
% This file is provided as a supplement to: Plett, Gregory L., "Battery
% Management Systems, Volume I, Battery Modeling," Artech House, 2015.

function [vk,irkc,zkc,OCV] = cellmodel(T,deltaT,iR0, zkp,irkp, cell_model,ik, Qgain)
  % Force data to be column vector(s)
  
%   ik=[DYNData.script1.current(round(t*10)),DYNData.script1.current(round(t*10)+1)];
%   ik=interp1(0.1*(1:length(DYNData.script1.current)),DYNData.script1.current,t,'nearest');
  ik = ik(:); iR0 = iR0(:);
  
  % Get model parameters from model structure
  RCfact = exp(-deltaT./abs(getParamESC('RCParam',T,cell_model)))';
  Q = Qgain* getParamESC('QParam',T,cell_model);
  RParam = getParamESC('RParam',T,cell_model);
  R0Param = getParamESC('R0Param',T,cell_model);
  etaParam = getParamESC('etaParam',T,cell_model);
  
  etaik = ik; 
  for iii=1:length(ik)
    if etaik(iii)<0
        etaik(iii) = etaParam*ik(iii); % compensate for coulombic efficiency
    end
  end
  % Simulate the dynamic states of the model
  %if exist('ss','file'), % use control-system-toolbox method, if available
%     sysd= ss(diag(RCfact),1-RCfact,eye(length(RCfact)),0,0.1);
%     irk = lsim(sysd,etaik,[],iR0);
  %else
    irkc = RCfact.*irkp + (1-RCfact)*etaik(1);
  %end
%    irkc2 = irk(2,:)';
%    irkc=(irkc1+irkc2)/2;
  zkc = zkp-etaik(1)*deltaT/(Q*3600); 

    
  % Compute output equation
  OCV = OCVfromSOCtemp(zkc,T,cell_model);
  vk = OCV - RParam*irkc - ik(1).*R0Param ;%+ M*hk + M0*sik;
  
  


function theParam = getParamESC(paramName,temp,model)
%   theFields = fields(model); % get list of fields stored in model
%   match = strcmpi(paramName,theFields); % see if any match desired data
%   if ~match, % if not, throw an error
%     error('Parameter "%s" does not exist in model',paramName);
%   end
%   fieldName = char(theFields(match)); % case-sensitive field name

  % if model contains data at only one temperature
  if isscalar(model.temps),
    if model.temps ~= temp, % check whether requested data exists
      error('Model does not contain requested data at this temperature');
    end
    theParam = model.(paramName);
    return
  end

  % Otherwise, model has multiple temperatures. Bound input "temp" between
  % mininum and maximum stored temperature to prohibit "NaN" in output
  theParamData = model.(paramName);
  temp = max(min(temp,max(model.temps)),min(model.temps)); 
  ind = find(model.temps == temp); % see if there is an exact match to
  if ~isempty(ind), % avoid call to (slow) interp1 whenever possible
    if size(theParamData,1) == 1,
      theParam = theParamData(ind);
    else
      theParam = theParamData(ind,:);
    end
  else % if there is not an exact match, we interpolate between parameter
    theParam = interp1(model.temps,theParamData,temp,'spline'); % values
  end  % stored at different temperatures
  
  % function ocv = OCVfromSOCtemp(soc,temp,model)
%
% Computes the fully rested open-circuit voltage for a particular state of 
% charge and temperature point
%
% Inputs: soc = scalar or matrix of cell state of charge points
%        temp = scalar or matrix of temperatures at which to calc. OCV
%       model = data structure produced by processDynamic
% Output: ocv = scalar or matrix of open circuit voltages -- one for every
%               soc and temperature input point

% Copyright (c) 2015 by Gregory L. Plett of the University of Colorado 
% Colorado Springs (UCCS). This work is licensed under a Creative Commons 
% Attribution-NonCommercial-ShareAlike 4.0 Intl. License, v. 1.0.
% It is provided "as is", without express or implied warranty, for 
% educational and informational purposes only.
%
% This file is provided as a supplement to: Plett, Gregory L., "Battery
% Management Systems, Volume I, Battery Modeling," Artech House, 2015.

function ocv=OCVfromSOCtemp(soc,temp,model)
  soccol = soc(:); % force soc to be column vector
  SOC = model.SOC(:); % force to be column vector
  OCV0 = model.OCV0(:); % force to be column vector
  OCVrel = model.OCVrel(:); % force to be column vector
  if isscalar(temp), % replicate a scalar temperature for all socs
    tempcol = temp*ones(size(soccol)); 
  else
    tempcol = temp(:); % force matrix temperature to be column vector
    if ~isequal(size(tempcol),size(soccol)),
      error(['Function inputs "soc" and "temp" must either have same '...
        'number of elements, or "temp" must be a scalar']);
    end
  end
  diffSOC=SOC(2)-SOC(1); % spacing between SOC points - assume uniform
  ocv=zeros(size(soccol)); % initialize output to zero
  I1=find(soccol <= SOC(1)); % indices of socs below model-stored data
  I2=find(soccol >= SOC(end)); % and of socs above model-stored data
  I3=find(soccol > SOC(1) & soccol < SOC(end)); % the rest of them
  I6=isnan(soccol); % if input is "not a number" for any locations

  % for voltages less than lowest stored soc datapoint, extrapolate off 
  % low end of table 
  if ~isempty(I1),
    dv = (OCV0(2)+tempcol.*OCVrel(2)) - (OCV0(1)+tempcol.*OCVrel(1));
    ocv(I1)= (soccol(I1)-SOC(1)).*dv(I1)/diffSOC + ...
             OCV0(1)+tempcol(I1).*OCVrel(1);
  end

  % for voltages greater than highest stored soc datapoint, extrapolate off
  % high end of table
  if ~isempty(I2),
    dv = (OCV0(end)+tempcol.*OCVrel(end)) - ...
         (OCV0(end-1)+tempcol.*OCVrel(end-1));
    ocv(I2) = (soccol(I2)-SOC(end)).*dv(I2)/diffSOC + ...
              OCV0(end)+tempcol(I2).*OCVrel(end);
  end

  % for normal soc range, manually interpolate (10x faster than "interp1")
  I4=(soccol(I3)-SOC(1))/diffSOC; % using linear interpolation
  I5=floor(I4); I45 = I4-I5; omI45 = 1-I45;
  ocv(I3)=OCV0(I5+1).*omI45 + OCV0(I5+2).*I45;
  ocv(I3)=ocv(I3) + tempcol(I3).*(OCVrel(I5+1).*omI45 + OCVrel(I5+2).*I45);
  ocv(I6)=0; % replace NaN SOCs with zero voltage
  ocv = reshape(ocv,size(soc)); % output is same shape as input

== matlab function sim_battery_pack_simulink_18_11/SCM3/cell8/cell_model ==
  data: vk output size=1; T input; deltaT input; iR0 input; zkp input; irkp input; irkc output size=3; zkc output size=1; OCV output size=1; cell_model parameter; ik input; Qgain parameter

% function [vk,irk,hk,zk,sik,OCV] = simCell(ik,T,deltaT,model,z0,iR0,h0)
% 
% Simulates an ESC model for input current ik at temperature T
%
% Inputs:  ik - current, where (+) is discharge
%          T  - temperature (degC)
%      deltaT - sampling interval in data (s)
%       model - standard model structure
%          z0 - initial cell state of charge
%         iR0 - initial resistor currents as column vector
%          h0 - initial hysteresis state
% Outputs: vk - cell voltage for all timesteps
%         irk - resistor currents (in R-C branches) for all timesteps
%          hk - hysteresis states for all timesteps
%          zk - state of charge for all timesteps
%         sik - instantaneous hysteresis for all timesteps
%         OCV - open-circuit voltage for all timesteps

% Copyright (c) 2015 by Gregory L. Plett of the University of Colorado 
% Colorado Springs (UCCS). This work is licensed under a Creative Commons 
% Attribution-NonCommercial-ShareAlike 4.0 Intl. License, v. 1.0.
% It is provided "as is", without express or implied warranty, for 
% educational and informational purposes only.
%
% This file is provided as a supplement to: Plett, Gregory L., "Battery
% Management Systems, Volume I, Battery Modeling," Artech House, 2015.

function [vk,irkc,zkc,OCV] = cellmodel(T,deltaT,iR0, zkp,irkp, cell_model,ik, Qgain)
  % Force data to be column vector(s)
  
%   ik=[DYNData.script1.current(round(t*10)),DYNData.script1.current(round(t*10)+1)];
%   ik=interp1(0.1*(1:length(DYNData.script1.current)),DYNData.script1.current,t,'nearest');
  ik = ik(:); iR0 = iR0(:);
  
  % Get model parameters from model structure
  RCfact = exp(-deltaT./abs(getParamESC('RCParam',T,cell_model)))';
  Q = Qgain* getParamESC('QParam',T,cell_model);
  RParam = getParamESC('RParam',T,cell_model);
  R0Param = getParamESC('R0Param',T,cell_model);
  etaParam = getParamESC('etaParam',T,cell_model);
  
  etaik = ik; 
  for iii=1:length(ik)
    if etaik(iii)<0
        etaik(iii) = etaParam*ik(iii); % compensate for coulombic efficiency
    end
  end
  % Simulate the dynamic states of the model
  %if exist('ss','file'), % use control-system-toolbox method, if available
%     sysd= ss(diag(RCfact),1-RCfact,eye(length(RCfact)),0,0.1);
%     irk = lsim(sysd,etaik,[],iR0);
  %else
    irkc = RCfact.*irkp + (1-RCfact)*etaik(1);
  %end
%    irkc2 = irk(2,:)';
%    irkc=(irkc1+irkc2)/2;
  zkc = zkp-etaik(1)*deltaT/(Q*3600); 

    
  % Compute output equation
  OCV = OCVfromSOCtemp(zkc,T,cell_model);
  vk = OCV - RParam*irkc - ik(1).*R0Param ;%+ M*hk + M0*sik;
  
  


function theParam = getParamESC(paramName,temp,model)
%   theFields = fields(model); % get list of fields stored in model
%   match = strcmpi(paramName,theFields); % see if any match desired data
%   if ~match, % if not, throw an error
%     error('Parameter "%s" does not exist in model',paramName);
%   end
%   fieldName = char(theFields(match)); % case-sensitive field name

  % if model contains data at only one temperature
  if isscalar(model.temps),
    if model.temps ~= temp, % check whether requested data exists
      error('Model does not contain requested data at this temperature');
    end
    theParam = model.(paramName);
    return
  end

  % Otherwise, model has multiple temperatures. Bound input "temp" between
  % mininum and maximum stored temperature to prohibit "NaN" in output
  theParamData = model.(paramName);
  temp = max(min(temp,max(model.temps)),min(model.temps)); 
  ind = find(model.temps == temp); % see if there is an exact match to
  if ~isempty(ind), % avoid call to (slow) interp1 whenever possible
    if size(theParamData,1) == 1,
      theParam = theParamData(ind);
    else
      theParam = theParamData(ind,:);
    end
  else % if there is not an exact match, we interpolate between parameter
    theParam = interp1(model.temps,theParamData,temp,'spline'); % values
  end  % stored at different temperatures
  
  % function ocv = OCVfromSOCtemp(soc,temp,model)
%
% Computes the fully rested open-circuit voltage for a particular state of 
% charge and temperature point
%
% Inputs: soc = scalar or matrix of cell state of charge points
%        temp = scalar or matrix of temperatures at which to calc. OCV
%       model = data structure produced by processDynamic
% Output: ocv = scalar or matrix of open circuit voltages -- one for every
%               soc and temperature input point

% Copyright (c) 2015 by Gregory L. Plett of the University of Colorado 
% Colorado Springs (UCCS). This work is licensed under a Creative Commons 
% Attribution-NonCommercial-ShareAlike 4.0 Intl. License, v. 1.0.
% It is provided "as is", without express or implied warranty, for 
% educational and informational purposes only.
%
% This file is provided as a supplement to: Plett, Gregory L., "Battery
% Management Systems, Volume I, Battery Modeling," Artech House, 2015.

function ocv=OCVfromSOCtemp(soc,temp,model)
  soccol = soc(:); % force soc to be column vector
  SOC = model.SOC(:); % force to be column vector
  OCV0 = model.OCV0(:); % force to be column vector
  OCVrel = model.OCVrel(:); % force to be column vector
  if isscalar(temp), % replicate a scalar temperature for all socs
    tempcol = temp*ones(size(soccol)); 
  else
    tempcol = temp(:); % force matrix temperature to be column vector
    if ~isequal(size(tempcol),size(soccol)),
      error(['Function inputs "soc" and "temp" must either have same '...
        'number of elements, or "temp" must be a scalar']);
    end
  end
  diffSOC=SOC(2)-SOC(1); % spacing between SOC points - assume uniform
  ocv=zeros(size(soccol)); % initialize output to zero
  I1=find(soccol <= SOC(1)); % indices of socs below model-stored data
  I2=find(soccol >= SOC(end)); % and of socs above model-stored data
  I3=find(soccol > SOC(1) & soccol < SOC(end)); % the rest of them
  I6=isnan(soccol); % if input is "not a number" for any locations

  % for voltages less than lowest stored soc datapoint, extrapolate off 
  % low end of table 
  if ~isempty(I1),
    dv = (OCV0(2)+tempcol.*OCVrel(2)) - (OCV0(1)+tempcol.*OCVrel(1));
    ocv(I1)= (soccol(I1)-SOC(1)).*dv(I1)/diffSOC + ...
             OCV0(1)+tempcol(I1).*OCVrel(1);
  end

  % for voltages greater than highest stored soc datapoint, extrapolate off
  % high end of table
  if ~isempty(I2),
    dv = (OCV0(end)+tempcol.*OCVrel(end)) - ...
         (OCV0(end-1)+tempcol.*OCVrel(end-1));
    ocv(I2) = (soccol(I2)-SOC(end)).*dv(I2)/diffSOC + ...
              OCV0(end)+tempcol(I2).*OCVrel(end);
  end

  % for normal soc range, manually interpolate (10x faster than "interp1")
  I4=(soccol(I3)-SOC(1))/diffSOC; % using linear interpolation
  I5=floor(I4); I45 = I4-I5; omI45 = 1-I45;
  ocv(I3)=OCV0(I5+1).*omI45 + OCV0(I5+2).*I45;
  ocv(I3)=ocv(I3) + tempcol(I3).*(OCVrel(I5+1).*omI45 + OCVrel(I5+2).*I45);
  ocv(I6)=0; % replace NaN SOCs with zero voltage
  ocv = reshape(ocv,size(soc)); % output is same shape as input
